simulink model "testFahrt"  (R2017a)
settings: Solver=FixedStepAuto  StartTime=0.0  StopTime=10  FixedStep=1/1000  RelTol=1e-3
values from neighbouring files (symbols this model uses):
  l_a = 0.184    [Kippreglerauslegung.m]    (also in Minv.m = 0.14; Roboterdaten.m = 0.14)
  r = 0.05    [Kippreglerauslegung.m]    (also in Minv.m; Roboterdaten.m)
  s = tf('s')    [Kippregler.m]    (also in Kippreglerauslegung.m; ahaaa.m)
libraries: slctrlblks x3, simulink x2, vrlib x1
settings Model: Creator=Stephan  LastModifiedBy=Timo

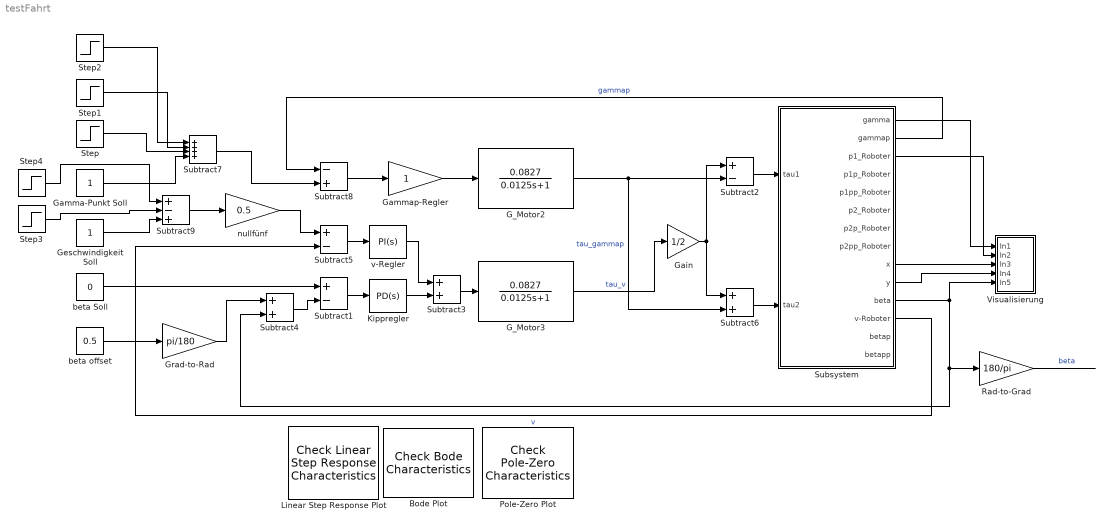
== system testFahrt ==
  Bode Plot : slctrlblks/Model Verification/Check Bode  Characteristics  InstantiateOnLoad=on  SaveOperatingPoints=off  LinearizationIOs={'/Geschwindigkeit Soll', 1, 'in', 'off', '';'/Subsystem', 12, 'out', 'off', ''}  LinearizeAt=SnapshotTimes  SnapshotTimes=[0]  TriggerType=rising  SampleTime=auto  RateConversionMethod=zoh  PreWarpFreq=10  UseExactDelayModel=off  UseFullBlockNameLabels=off  UseBusSignalLabels=off  enabled=on  stopWhenAssertionFail=off  export=off  ViewDlgPos=[311 383 510 390]  OpenViewOnLoad=off  LaunchViewOnOpen=on  FrequencyUnits=rad/s  MagnitudeUnits=dB  PhaseUnits=deg  TimeUnits=seconds  EnableUpperBound=off  UpperBoundFrequencies=[]  UpperBoundMagnitudes=[]  EnableLowerBound=off  LowerBoundFrequencies=[]  LowerBoundMagnitudes=[]
      settings: SourceProductName=Simulink Control Design
  G_Motor2 : TransferFcn  Numerator=0.0827  Denominator=[0.0125 1]
  G_Motor3 : TransferFcn  Numerator=0.0827  Denominator=[0.0125 1]
  Gain : Gain  Gain=1/2
  Gamma-Punkt Soll : Constant
  Gammap-Regler : Gain
  Geschwindigkeit Soll : Constant
  Grad-to-Rad : Gain  Gain=pi/180
  Kippregler : simulink/Continuous/PID Controller  Controller=PD  TimeDomain=Continuous-time  SampleTime=-1  IntegratorMethod=Forward Euler  FilterMethod=Forward Euler  Form=Parallel  UseFilter=on  ControllerParametersSource=internal  P=-1.562*12.09  I=0  D=-0.11*12.09  N=1000  InitialConditionSource=internal  InitialConditionForIntegrator=0  InitialConditionForFilter=0  ExternalReset=none  LimitOutput=off  UpperSaturationLimit=inf  LowerSaturationLimit=-inf  LinearizeAsGain=on  AntiWindupMode=none  Kb=1  TrackingMode=off  Kt=1  PParamMin=[]  PParamMax=[]  IParamMin=[]  IParamMax=[]  DParamMin=[]  DParamMax=[]  NParamMin=[]  NParamMax=[]  KbParamMin=[]  KbParamMax=[]  KtParamMin=[]  KtParamMax=[]  POutMin=[]  POutMax=[]  IOutMin=[]  IOutMax=[]  DOutMin=[]  DOutMax=[]  NOutMin=[]  NOutMax=[]  KbOutMin=[]  KbOutMax=[]  KtOutMin=[]  KtOutMax=[]  IntegratorOutMin=[]  IntegratorOutMax=[]  FilterOutMin=[]  FilterOutMax=[]  SumOutMin=[]  SumOutMax=[]  SumI1OutMin=[]  SumI1OutMax=[]  SumI2OutMin=[]  SumI2OutMax=[]  SumI3OutMin=[]  SumI3OutMax=[]  SumDOutMin=[]  SumDOutMax=[]  SaturationOutMin=[]  SaturationOutMax=[]  IntegratorContinuousStateAttributes=''  IntegratorStateMustResolveToSignalObject=off  IntegratorRTWStateStorageClass=Auto  FilterContinuousStateAttributes=''  FilterStateMustResolveToSignalObject=off  FilterRTWStateStorageClass=Auto  DifferentiatorICPrevScaledInput=0  DifferentiatorOutMin=[]  DifferentiatorOutMax=[]  InitialConditionSetting=State (most efficient)
  Linear Step Response Plot : slctrlblks/Model Verification/Check Linear Step Response Characteristics  InstantiateOnLoad=on  SaveOperatingPoints=off  LinearizationIOs={'/Geschwindigkeit Soll', 1, 'in', 'off', '';'/Subsystem', 12, 'out', 'off', ''}  LinearizeAt=SnapshotTimes  SnapshotTimes=[0]  TriggerType=rising  SampleTime=auto  RateConversionMethod=zoh  PreWarpFreq=10  UseExactDelayModel=off  UseFullBlockNameLabels=off  UseBusSignalLabels=off  enabled=on  stopWhenAssertionFail=off  export=off  ViewDlgPos=[1 41 1920 963]  OpenViewOnLoad=off  LaunchViewOnOpen=on  FrequencyUnits=rad/s  MagnitudeUnits=dB  PhaseUnits=deg  TimeUnits=seconds  EnableStepResponseBound=off  FinalValue=[]  RiseTime=[]  PercentRise=[]  SettlingTime=[]  PercentSettling=[]  PercentOvershoot=[]  PercentUndershoot=[]
      settings: SourceProductName=Simulink Control Design  SourceProductBaseCode=SD  SaveToWorkspace=off  SaveName=sys
  Pole-Zero Plot : slctrlblks/Model Verification/Check Pole-Zero Characteristics  InstantiateOnLoad=on  SaveOperatingPoints=off  LinearizationIOs={'/Geschwindigkeit Soll', 1, 'in', 'off', '';'/Subsystem', 12, 'out', 'off', ''}  LinearizeAt=SnapshotTimes  SnapshotTimes=[0]  TriggerType=rising  SampleTime=auto  RateConversionMethod=zoh  PreWarpFreq=10  UseExactDelayModel=off  UseFullBlockNameLabels=off  UseBusSignalLabels=off  enabled=on  stopWhenAssertionFail=off  export=off  ViewDlgPos=[1031 452 510 390]  LaunchViewOnOpen=on  OpenViewOnLoad=off  FrequencyUnits=rad/s  MagnitudeUnits=dB  PhaseUnits=deg  TimeUnits=seconds  EnableSettlingTime=off  SettlingTime=[]  EnablePercentOvershoot=off  PercentOvershoot=[]  EnableDampingRatio=off  DampingRatio=[]  EnableNaturalFrequency=off  NaturalFrequencyBound=>=  NaturalFrequency=[]
      settings: SourceProductName=Simulink Control Design  SourceProductBaseCode=SD  SaveToWorkspace=off  SaveName=sys
  Rad-to-Grad : Gain  Gain=180/pi
  Step : Step  After=-2  SampleTime=0
  Step1 : Step  Time=3  SampleTime=0
  Step2 : Step  Time=5  SampleTime=0
  Step3 : Step  Time=3  After=2  SampleTime=0
  Step4 : Step  Time=6  SampleTime=0
  Subsystem : Subsystem
  Subtract1 : Sum  Inputs=+-
  Subtract2 : Sum  Inputs=+-
  Subtract3 : Sum
  Subtract4 : Sum
  Subtract5 : Sum  Inputs=+-
  Subtract6 : Sum
  Subtract7 : Sum  Inputs=++++
  Subtract8 : Sum  Inputs=-+
  Subtract9 : Sum  Inputs=+-+
  Visualisierung : Subsystem
  beta Soll : Constant  Value=0
  beta offset : Constant  Value=0.5
  nullfünf : Gain  Gain=0.5
  v-Regler : simulink/Continuous/PID Controller  Controller=PI  TimeDomain=Continuous-time  SampleTime=-1  IntegratorMethod=Forward Euler  FilterMethod=Forward Euler  Form=Parallel  UseFilter=on  ControllerParametersSource=internal  P=-0.5*12.09  I=-0.5*12.09  D=0.003  N=1000  InitialConditionSource=internal  InitialConditionForIntegrator=0  InitialConditionForFilter=0  ExternalReset=none  LimitOutput=off  UpperSaturationLimit=inf  LowerSaturationLimit=-inf  LinearizeAsGain=on  AntiWindupMode=none  Kb=1  TrackingMode=off  Kt=1  PParamMin=[]  PParamMax=[]  IParamMin=[]  IParamMax=[]  DParamMin=[]  DParamMax=[]  NParamMin=[]  NParamMax=[]  KbParamMin=[]  KbParamMax=[]  KtParamMin=[]  KtParamMax=[]  POutMin=[]  POutMax=[]  IOutMin=[]  IOutMax=[]  DOutMin=[]  DOutMax=[]  NOutMin=[]  NOutMax=[]  KbOutMin=[]  KbOutMax=[]  KtOutMin=[]  KtOutMax=[]  IntegratorOutMin=[]  IntegratorOutMax=[]  FilterOutMin=[]  FilterOutMax=[]  SumOutMin=[]  SumOutMax=[]  SumI1OutMin=[]  SumI1OutMax=[]  SumI2OutMin=[]  SumI2OutMax=[]  SumI3OutMin=[]  SumI3OutMax=[]  SumDOutMin=[]  SumDOutMax=[]  SaturationOutMin=[]  SaturationOutMax=[]  IntegratorContinuousStateAttributes=''  IntegratorStateMustResolveToSignalObject=off  IntegratorRTWStateStorageClass=Auto  FilterContinuousStateAttributes=''  FilterStateMustResolveToSignalObject=off  FilterRTWStateStorageClass=Auto  DifferentiatorICPrevScaledInput=0  DifferentiatorOutMin=[]  DifferentiatorOutMax=[]  InitialConditionSetting=State (most efficient)
  wires:
  Subsystem/11(beta) -> Visualisierung/5(In5), Subtract4/2, Rad-to-Grad/1
  Gammap-Regler/1 -> G_Motor2/1
  Subsystem/2(gammap) -> Subtract8/1  "gammap"
  Gamma-Punkt Soll/1 -> Subtract7/4
  Gain/1 -> Subtract6/1, Subtract2/1
  G_Motor3/1 -> Gain/1  "tau_v"
  Subtract6/1 -> Subsystem/2(tau2)
  G_Motor2/1 -> Subtract2/2, Subtract6/2  "tau_gammap"
  Subtract2/1 -> Subsystem/1(tau1)
  Subtract1/1 -> Kippregler/1
  beta Soll/1 -> Subtract1/1
  Geschwindigkeit Soll/1 -> Subtract9/3
  Subtract8/1 -> Gammap-Regler/1
  Subsystem/12(v-Roboter) -> Subtract5/2  "v"
  Subsystem/1(gamma) -> Visualisierung/1(In1)
  Subsystem/3(p1_Roboter) -> Visualisierung/2(In2)
  Subsystem/9(x) -> Visualisierung/3(In3)
  Subsystem/10(y) -> Visualisierung/4(In4)
  Subtract5/1 -> v-Regler/1
  Subtract3/1 -> G_Motor3/1
  Kippregler/1 -> Subtract3/2
  Rad-to-Grad/1 -> ?  "beta"
  beta offset/1 -> Grad-to-Rad/1
  Subtract4/1 -> Subtract1/2
  Grad-to-Rad/1 -> Subtract4/1
  v-Regler/1 -> Subtract3/1
  Subtract7/1 -> Subtract8/2
  Step/1 -> Subtract7/3
  Step1/1 -> Subtract7/2
  Step2/1 -> Subtract7/1
  Subtract9/1 -> nullfünf/1
  Step3/1 -> Subtract9/2
  Step4/1 -> Subtract9/1
  nullfünf/1 -> Subtract5/1

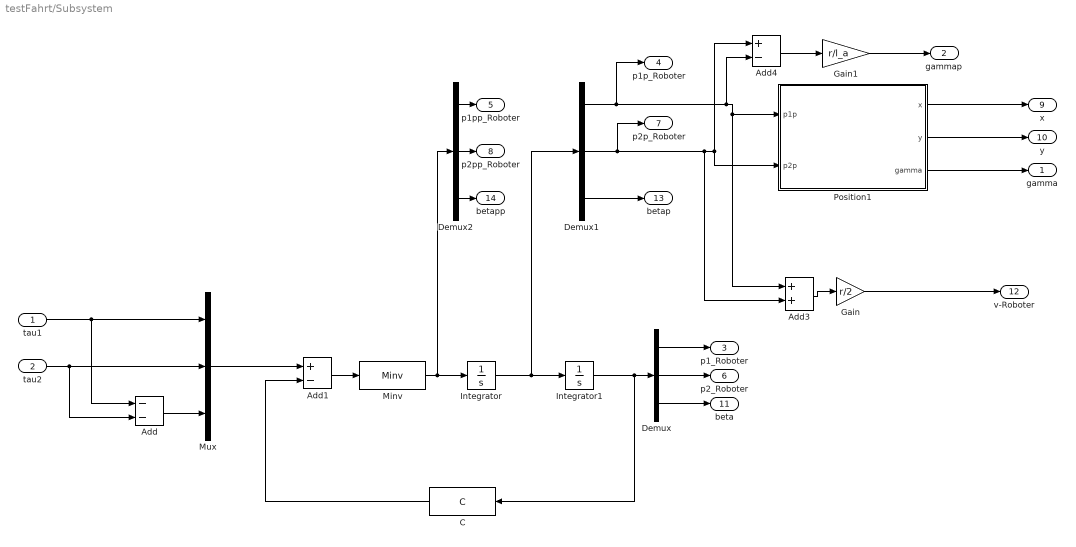
== system testFahrt/Subsystem ==
  tau1 : Inport
  tau2 : Inport  Port=2
  Add : Sum  Inputs=--
  Add1 : Sum  Inputs=+-
  Add3 : Sum
  Add4 : Sum  Inputs=+-
  C : MATLABFcn  MATLABFcn=C  OutputDimensions=3
  Demux : Demux  Outputs=3
  Demux1 : Demux  Outputs=3
  Demux2 : Demux  Outputs=3
  Gain : Gain  Gain=r/2
  Gain1 : Gain  Gain=r/l_a
  Integrator : Integrator
  Integrator1 : Integrator
  Minv : MATLABFcn  MATLABFcn=Minv  OutputDimensions=3
  Mux : Mux  Inputs=3
  Position1 : Subsystem
  gamma : Outport
  gammap : Outport  Port=2
  p1_Roboter : Outport  Port=3
  p1p_Roboter : Outport  Port=4
  p1pp_Roboter : Outport  Port=5
  p2_Roboter : Outport  Port=6
  p2p_Roboter : Outport  Port=7
  p2pp_Roboter : Outport  Port=8
  x : Outport  Port=9
  y : Outport  Port=10
  beta : Outport  Port=11
  v-Roboter : Outport  Port=12
  betap : Outport  Port=13
  betapp : Outport  Port=14
  wires:
  tau1/1 -> Mux/1, Add/1
  tau2/1 -> Mux/2, Add/2
  Add/1 -> Mux/3
  Mux/1 -> Add1/1
  Integrator/1 -> Demux1/1, Integrator1/1
  Add1/1 -> Minv/1
  Integrator1/1 -> C/1, Demux/1
  Demux/1 -> p1_Roboter/1
  Demux/2 -> p2_Roboter/1
  Demux/3 -> beta/1
  Demux1/3 -> betap/1
  Demux1/2 -> p2p_Roboter/1, Add4/1, Position1/2(p2p), Add3/2
  Demux1/1 -> p1p_Roboter/1, Add4/2, Position1/1(p1p), Add3/1
  C/1 -> Add1/2
  Demux2/2 -> p2pp_Roboter/1
  Demux2/1 -> p1pp_Roboter/1
  Demux2/3 -> betapp/1
  Minv/1 -> Demux2/1, Integrator/1
  Add3/1 -> Gain/1
  Add4/1 -> Gain1/1
  Gain1/1 -> gammap/1
  Gain/1 -> v-Roboter/1
  Position1/1(x) -> x/1
  Position1/2(y) -> y/1
  Position1/3(gamma) -> gamma/1

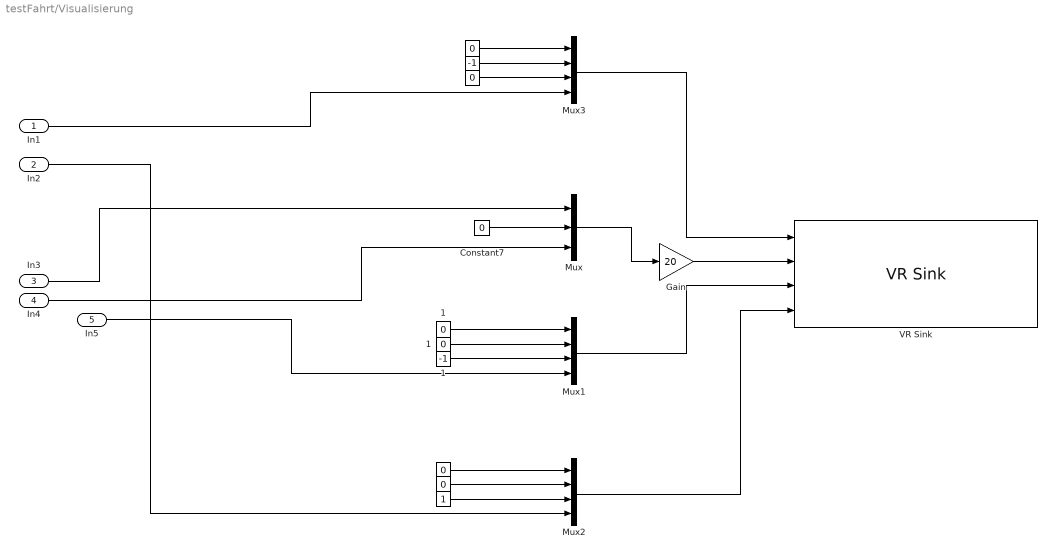
== system testFahrt/Visualisierung ==
  In1 : Inport
  In2 : Inport  Port=2
  In3 : Inport  Port=3
  In4 : Inport  Port=4
  In5 : Inport  Port=5
  "   " : Constant  Value=0
  "     " : Constant  Value=0
  "      " : Constant
  "               " : Constant  Value=0
  "                       " : Constant  Value=-1
  "                                " : Constant  Value=0
  "      1" : Constant  Value=-1
  "     1" : Constant  Value=0
  "   1" : Constant  Value=0
  Constant7 : Constant  Value=0
  Gain : Gain  Gain=20
  Mux : Mux  Inputs=3
  Mux1 : Mux
  Mux2 : Mux
  Mux3 : Mux
  VR Sink : vrlib/VR Sink  InstantiateOnLoad=on  SampleTime=0.1  ViewEnable=on  RemoteChange=off  RemoteView=off  FieldsWritten=SegwayPosition.rotation.4.1.1.double#SegwayPosition.translation.3.1.1.double#SegwayKippwinkel.rotation.4.1.1.double#Radmarkierungen.rotation.4.1.1.double  WorldFileName=SegwayWorldModell.wrl  WorldDescription=Straight Road Strip - 2 Lanes  AutoView=off  VideoDimensions=[]  AllowVariableSize=off  FigureProperties="{'Position', 'Name', 'Viewpoint', 'CameraBound', 'CameraDirection', 'CameraPosition', 'CameraUpVector', 'ZoomFactor', 'Antialiasing', 'Headlight', 'Lighting', 'NavPanel', 'Sound', 'StatusBar', 'Stereo3D', 'Stereo3DCameraOffset', 'Stereo3DHIT', 'ToolBar', 'Textures', 'Transparency', 'Triad', 'Wireframe', 'NavZones', 'NavMode', 'NavSpeed', 'CaptureFileFormat', 'CaptureFileName', 'Record2DCompressMethod', 'Record2DCompressQuality', 'Record2D', 'Record2DFileName', 'Record2DFPS'; [1.2470000000000000e+03   8.6000000000000000e+01   6.5400000000000000e+02   5.8900000000000000e+02], 'Straight Road Strip - 2 Lanes', 'Scene in YZ', 'on', [6.8878389074001345e-01  -7.2387705120185841e-01   3.9733696031681393e-02], [-1.1768220104021772e+02   1.3532201650487801e+02  -9.1998463838461149e+01], [7.1627692757399120e-01   6.8796542563424590e-01   1.1683722076909921e-01], [1.0000000000000000e+00], 'on', 'off', 'on', 'halfbar', 'on', 'on', 'off', [1.0000000149011612e-01], [0.0000000000000000e+00], 'on', 'on', 'on', 'none', 'off', 'off', 'examine', 'normal', 'tif', '%f_anim_%n.tif', 'auto', [7.5000000000000000e+01], 'off', '%f_anim_%n.avi', 'auto'}"
      settings: SourceProductBaseCode=VR
  wires:
  In3/1 -> Mux/1
  "     1"/1 -> Mux1/2
  "                       "/1 -> Mux3/2
  "   1"/1 -> Mux1/1
  "   "/1 -> Mux2/1
  In2/1 -> Mux2/4
  "      "/1 -> Mux2/3
  "               "/1 -> Mux3/3
  Mux1/1 -> VR Sink/3
  Mux2/1 -> VR Sink/4
  In1/1 -> Mux3/4
  "                                "/1 -> Mux3/1
  "      1"/1 -> Mux1/3
  Constant7/1 -> Mux/2
  In4/1 -> Mux/3
  Mux3/1 -> VR Sink/1
  "     "/1 -> Mux2/2
  Mux/1 -> Gain/1
  In5/1 -> Mux1/4
  Gain/1 -> VR Sink/2

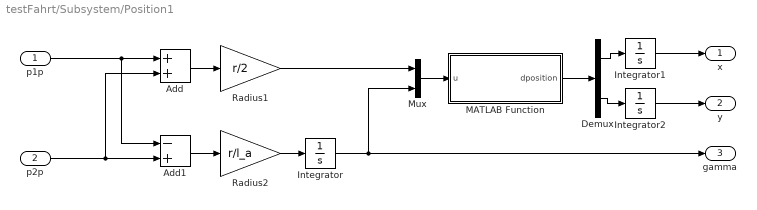
== system testFahrt/Subsystem/Position1 ==
  p1p : Inport
  p2p : Inport  Port=2
  Add : Sum
  Add1 : Sum  Inputs=-+
  Demux : Demux  Outputs=2
  Integrator : Integrator
  Integrator1 : Integrator
  Integrator2 : Integrator
  MATLAB Function : MATLAB Function  TreatAsAtomicUnit=on
  Mux : Mux  Inputs=2
  Radius1 : Gain  Gain=r/2
  Radius2 : Gain  Gain=r/l_a
  x : Outport
  y : Outport  Port=2
  gamma : Outport  Port=3
  wires:
  Add/1 -> Radius1/1
  p2p/1 -> Add/2, Add1/2
  Add1/1 -> Radius2/1
  p1p/1 -> Add1/1, Add/1
  Integrator/1 -> gamma/1, Mux/2
  Radius2/1 -> Integrator/1
  MATLAB Function/1(dposition) -> Demux/1
  Demux/1 -> Integrator1/1
  Integrator1/1 -> x/1
  Demux/2 -> Integrator2/1
  Integrator2/1 -> y/1
  Radius1/1 -> Mux/1
  Mux/1 -> MATLAB Function/1(u)

== matlab function testFahrt/Subsystem/Position1/MATLAB Function ==
  data: u input; dposition output
function dposition  = fcn(u)

dx = u(1);
gamma = u(2);

dposition = dx*[cos(gamma); sin(gamma)];
